simulink model "Control_System"  (R2018a)
settings: Solver=VariableStepAuto  StartTime=0.0  StopTime=10  RelTol=1e-3
libraries: simulink x1
settings Model: Creator=11011726  LastModifiedBy=11011726

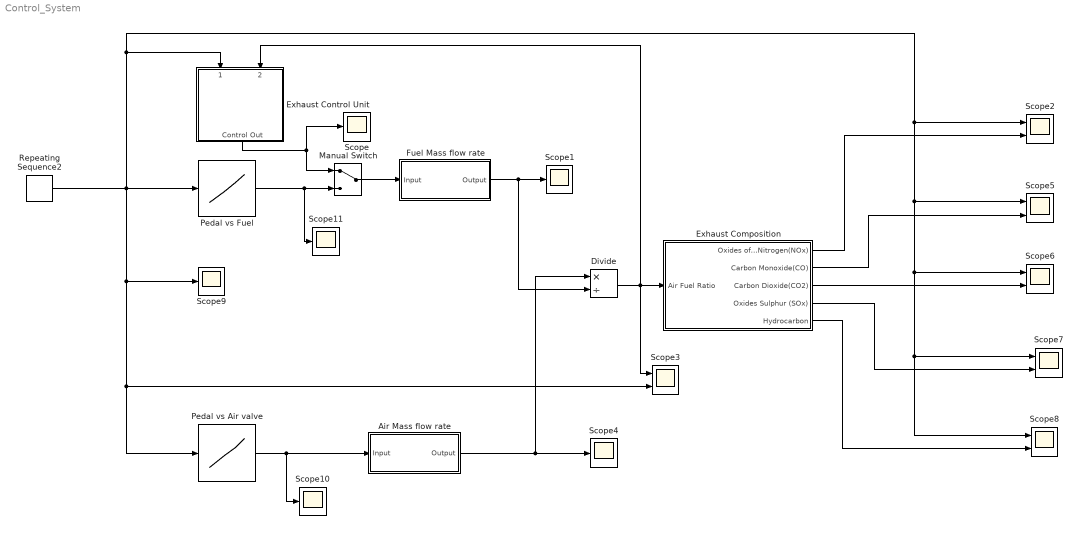
== system Control_System ==
  Air Mass flow rate : Subsystem
  Divide : Product  Inputs=*/
  "Exhaust Composition " : Subsystem
  Exhaust Control Unit : Subsystem
  Fuel Mass flow rate : Subsystem
  Manual Switch : ManualSwitch
  Pedal vs Air valve : Lookup_n-D  NumberOfTableDimensions=1  BreakpointsForDimension1=[0.1 0.5 1 2 5 7 10]  Table=|  InternalRulePriority=Speed  RndMeth=Simplest  InputSameDT=on
      | [1
      | 15
      | 10
      | 20
      | 50
      | 70
      | 100]
  Pedal vs Fuel : Lookup_n-D  NumberOfTableDimensions=1  BreakpointsForDimension1=[0.1 0.5 1 2 5 7 10]  BreakpointsForDimension1FirstPoint=5.4517133956386  Table=|  InternalRulePriority=Speed  RndMeth=Simplest  InputSameDT=on
      | [0.48
      | 15
      | 20
      | 18
      | 50
      | 65
      | 100]
  Repeating Sequence2 : simulink/Sources/Repeating Sequence  rep_seq_t=|  rep_seq_y=|
      rep_seq_t=|
      | [0
      | 0.5
      | 1
      | 1.5
      | 2
      | 2.5
      | 3
      | 3.5
      | 4
      | 4.5
      | 5]
      rep_seq_y=|
      | [1
      | 5
      | 2
      | 4
      | 7
      | 10
      | 10
      | 5
      | 2
      | 4
      | 7]
  Scope{,1,4,9..11} (6 alike) : Scope
  Scope{2..3,5..8} (6 alike) : Scope  NumInputPorts=2
  wires:
  Pedal vs Fuel/1 -> Scope11/1, Manual Switch/2
  Exhaust Control Unit/1(Control Out) -> Scope/1, Manual Switch/1
  Manual Switch/1 -> Fuel Mass flow rate/1(Input)
  Pedal vs Air valve/1 -> Scope10/1, Air Mass flow rate/1(Input)
  Fuel Mass flow rate/1("Output ") -> Scope1/1, Divide/2
  Air Mass flow rate/1(Output) -> Scope4/1, Divide/1
  Repeating Sequence2/1 -> Scope8/1, Scope7/1, Scope6/1, Scope5/1, Scope2/1, Exhaust Control Unit/1(Accelarator Input), Scope9/1, Pedal vs Air valve/1, Scope3/2, Pedal vs Fuel/1
  Divide/1 -> Exhaust Control Unit/2(Air/Fuel Ration), "Exhaust Composition "/1(Air Fuel Ratio), Scope3/1
  "Exhaust Composition "/2(Carbon Monoxide(CO)) -> Scope5/2
  "Exhaust Composition "/1(Oxides of Nitrogen(NOx)) -> Scope2/2
  "Exhaust Composition "/3(Carbon Dioxide(CO2)) -> Scope6/2
  "Exhaust Composition "/4(Oxides Sulphur (SOx)) -> Scope7/2
  "Exhaust Composition "/5(Hydrocarbon) -> Scope8/2

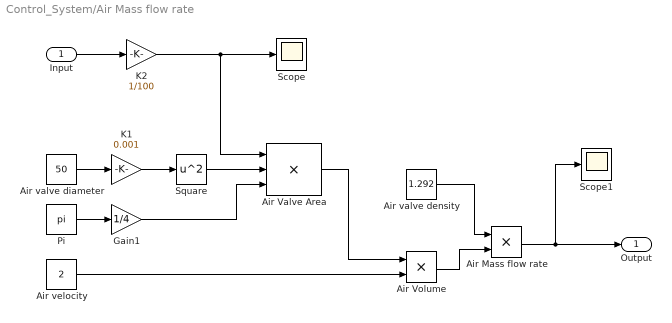
== system Control_System/Air Mass flow rate ==
  Input : Inport
  Air Mass flow rate : Product
  Air Valve Area : Product  Inputs=3
  Air Volume : Product
  Air valve density : Constant  Value=1.292
  Air valve diameter : Constant  Value=50
  Air velocity : Constant  Value=2
  Gain1 : Gain  Gain=1/4
  K1 : Gain  Gain=0.001
  K2 : Gain  Gain=1/100
  Pi : Constant  Value=pi
  Scope : Scope
  Scope1 : Scope
  Square : Math  Operator=square  SaturateOnIntegerOverflow=on
  Output : Outport
  wires:
  Input/1 -> K2/1
  Gain1/1 -> Air Valve Area/3
  Square/1 -> Air Valve Area/2
  Air Valve Area/1 -> Air Volume/1
  Pi/1 -> Gain1/1
  Air velocity/1 -> Air Volume/2
  K2/1 -> Scope/1, Air Valve Area/1
  Air Volume/1 -> Air Mass flow rate/2
  Air Mass flow rate/1 -> Scope1/1, Output/1
  Air valve density/1 -> Air Mass flow rate/1
  Air valve diameter/1 -> K1/1
  K1/1 -> Square/1

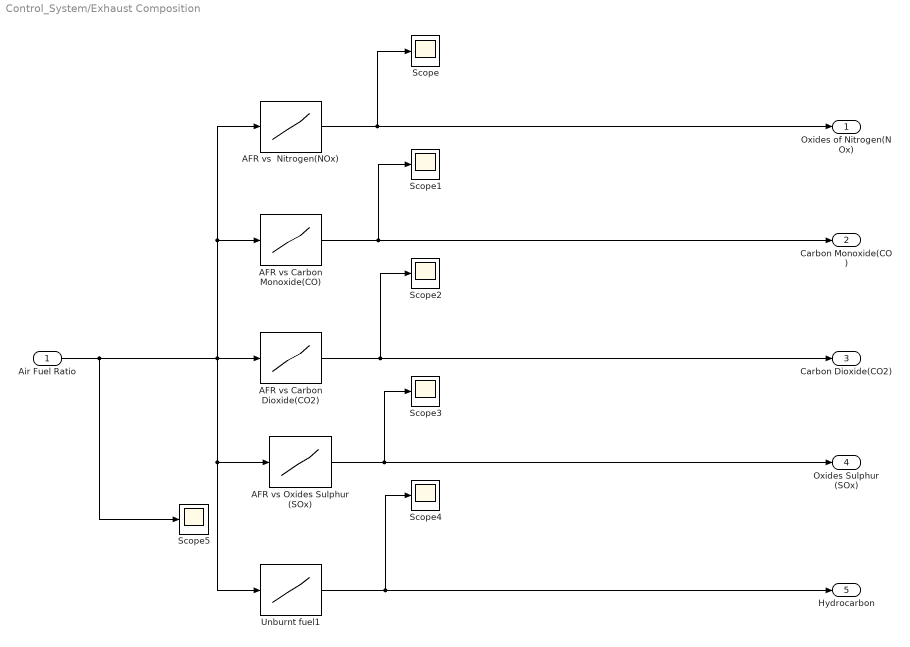
== system Control_System/Exhaust Composition  ==
  Air Fuel Ratio : Inport
  " AFR vs Carbon Monoxide(CO)" : Lookup_n-D  NumberOfTableDimensions=1  BreakpointsForDimension1=[10 14.5 14.6 14.7 14.8 15 15.5 18]  BreakpointsForDimension1FirstPoint=5.4517133956386  Table=[12 8 4 0.1 0.1 0.05 0.03 0.015]  InternalRulePriority=Speed  RndMeth=Simplest  InputSameDT=on
  "AFR vs  Nitrogen(NOx) " : Lookup_n-D  NumberOfTableDimensions=1  BreakpointsForDimension1=[10 14.5 14.6 14.7 14.8 15 15.5 18]  BreakpointsForDimension1FirstPoint=5.4517133956386  Table=[1 2.5 5 10 20 30 50 65]  InternalRulePriority=Speed  RndMeth=Simplest  InputSameDT=on
  AFR vs Carbon Dioxide(CO2) : Lookup_n-D  NumberOfTableDimensions=1  BreakpointsForDimension1=[10 14.5 14.6 14.7 14.8 15 15.5 18]  BreakpointsForDimension1FirstPoint=5.4517133956386  Table=[13 13 13.5 14 14 15 15 16]  InternalRulePriority=Speed  RndMeth=Simplest  InputSameDT=on
  AFR vs Oxides Sulphur (SOx) : Lookup_n-D  NumberOfTableDimensions=1  BreakpointsForDimension1=[10 14.5 14.6 14.7 14.8 15 15.5 18]  BreakpointsForDimension1FirstPoint=5.4517133956386  Table=[12 12 12.5 13 13 13 14 14]  InternalRulePriority=Speed  RndMeth=Simplest  InputSameDT=on
  Scope{,1..5} (6 alike) : Scope
  Unburnt fuel1 : Lookup_n-D  NumberOfTableDimensions=1  BreakpointsForDimension1=[10 14.1 14.5 14.6 14.7 14.8 15 15.5 18]  BreakpointsForDimension1FirstPoint=5.4517133956386  Table=[6 3 2 1.5 0 0 0 0 0]  InternalRulePriority=Speed  RndMeth=Simplest  InputSameDT=on
  Oxides of Nitrogen(NOx) : Outport
  Carbon Monoxide(CO) : Outport  Port=2
  Carbon Dioxide(CO2) : Outport  Port=3
  Oxides Sulphur (SOx) : Outport  Port=4
  Hydrocarbon : Outport  Port=5
  wires:
  Unburnt fuel1/1 -> Hydrocarbon/1, Scope4/1
  AFR vs Carbon Dioxide(CO2)/1 -> Scope2/1, Carbon Dioxide(CO2)/1
  AFR vs Oxides Sulphur (SOx)/1 -> Oxides Sulphur (SOx)/1, Scope3/1
  Air Fuel Ratio/1 -> "AFR vs  Nitrogen(NOx) "/1, " AFR vs Carbon Monoxide(CO)"/1, AFR vs Carbon Dioxide(CO2)/1, Unburnt fuel1/1, AFR vs Oxides Sulphur (SOx)/1, Scope5/1
  " AFR vs Carbon Monoxide(CO)"/1 -> Carbon Monoxide(CO)/1, Scope1/1
  "AFR vs  Nitrogen(NOx) "/1 -> Scope/1, Oxides of Nitrogen(NOx)/1

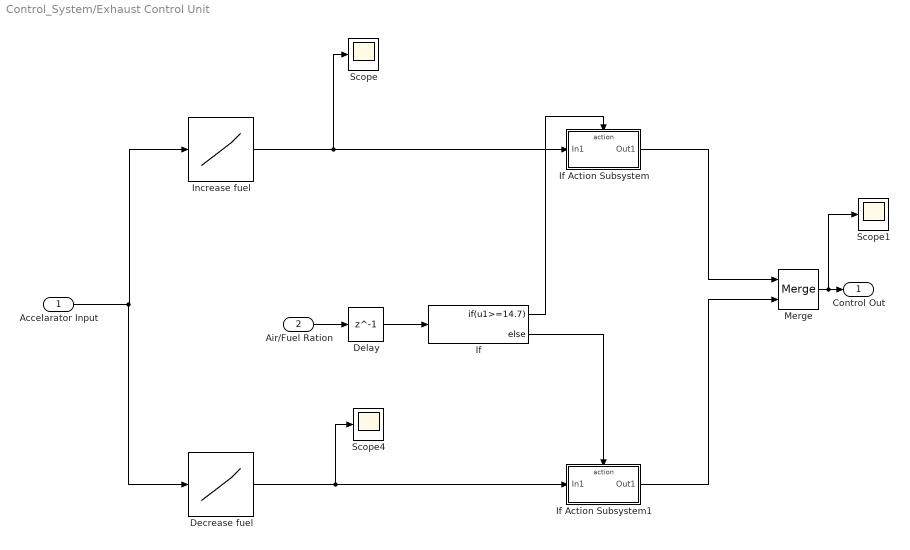
== system Control_System/Exhaust Control Unit ==
  Accelarator Input : Inport
  Air/Fuel Ration : Inport  Port=2
  Decrease fuel : Lookup_n-D  NumberOfTableDimensions=1  BreakpointsForDimension1=[0.1 0.5 1 2 5 7 10]  BreakpointsForDimension2=[1 7 10 14.7 16 20 40]  Table=|  InternalRulePriority=Speed  RndMeth=Simplest  InputSameDT=on
      | [0.5
      | 15
      | 20
      | 20
      | 50
      | 70
      | 100]
  Delay : Delay  DelayLength=1  InitialCondition=0
  If : If  IfExpression=u1>=14.7
  If Action Subsystem : Subsystem  TreatAsAtomicUnit=on
  If Action Subsystem1 : Subsystem  TreatAsAtomicUnit=on
  "Increase fuel " : Lookup_n-D  NumberOfTableDimensions=1  BreakpointsForDimension1=[0.1 0.5 1 2 5 7 10]  Table=|  InternalRulePriority=Speed  RndMeth=Simplest  InputSameDT=on
      | [0.5
      | 15
      | 20
      | 20
      | 50
      | 70
      | 100]
  Merge : Merge
  Scope : Scope
  Scope1 : Scope
  Scope4 : Scope
  Control Out : Outport
  wires:
  If/1 -> If Action Subsystem/Action
  If Action Subsystem1/1(Out1) -> Merge/2
  If Action Subsystem/1(Out1) -> Merge/1
  Accelarator Input/1 -> Decrease fuel/1, "Increase fuel "/1
  Air/Fuel Ration/1 -> Delay/1
  Delay/1 -> If/1
  Merge/1 -> Scope1/1, Control Out/1
  Decrease fuel/1 -> If Action Subsystem1/1(In1), Scope4/1
  "Increase fuel "/1 -> Scope/1, If Action Subsystem/1(In1)
  If/2 -> If Action Subsystem1/Action

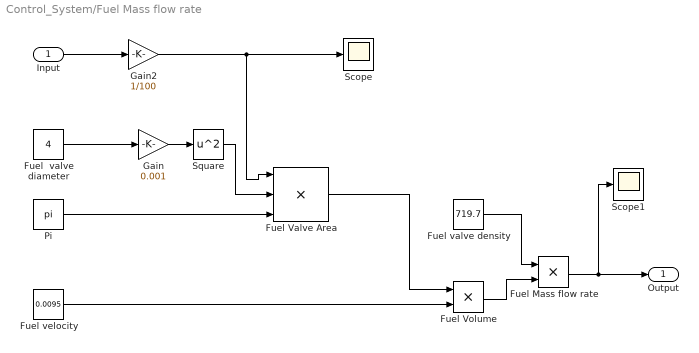
== system Control_System/Fuel Mass flow rate ==
  Input : Inport
  Fuel  valve diameter : Constant  Value=4
  Fuel Mass flow rate : Product
  Fuel Valve Area : Product  Inputs=3
  Fuel Volume : Product
  Fuel valve density : Constant  Value=719.7
  Fuel velocity : Constant  Value=0.0095
  Gain : Gain  Gain=0.001
  Gain2 : Gain  Gain=1/100
  Pi : Constant  Value=pi
  Scope : Scope
  Scope1 : Scope
  Square : Math  Operator=square  SaturateOnIntegerOverflow=on
  "Output " : Outport
  wires:
  Input/1 -> Gain2/1
  Pi/1 -> Fuel Valve Area/3
  Fuel  valve diameter/1 -> Gain/1
  Square/1 -> Fuel Valve Area/2
  Fuel Valve Area/1 -> Fuel Volume/1
  Fuel valve density/1 -> Fuel Mass flow rate/1
  Gain/1 -> Square/1
  Fuel Volume/1 -> Fuel Mass flow rate/2
  Gain2/1 -> Scope/1, Fuel Valve Area/1
  Fuel Mass flow rate/1 -> Scope1/1, "Output "/1
  Fuel velocity/1 -> Fuel Volume/2

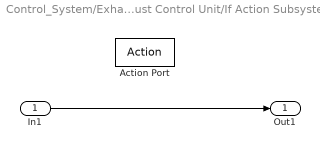
== system Control_System/Exhaust Control Unit/If Action Subsystem ==
  In1 : Inport
  Action Port : ActionPort  ActionType=then
  Out1 : Outport
  wires:
  In1/1 -> Out1/1

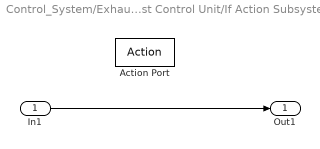
== system Control_System/Exhaust Control Unit/If Action Subsystem1 ==
  In1 : Inport
  Action Port : ActionPort  ActionType=else
  Out1 : Outport
  wires:
  In1/1 -> Out1/1
